simulink model "workshop_stateflow"  (R2020a)
settings: Solver=VariableStepAuto  StartTime=0.0  StopTime=inf  RelTol=1e-3
settings Model: Creator=matas  LastModifiedBy=matas

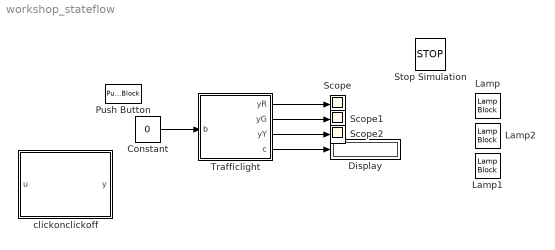
== system workshop_stateflow ==
  Constant : Constant  Value=0
  Display : Display
  Lamp : LampBlock
  Lamp1 : LampBlock
  Lamp2 : LampBlock
  Push Button : PushButtonBlock
  Scope : Scope
  Scope1 : Scope
  Scope2 : Scope
  Stop Simulation : Stop
  Trafficlight : Stateflow chart  TreatAsAtomicUnit=on
  clickonclickoff : Stateflow chart  TreatAsAtomicUnit=on
  wires:
  Constant/1 -> Trafficlight/1(b)
  Trafficlight/1(yR) -> Scope/1
  Trafficlight/2(yG) -> Scope1/1
  Trafficlight/3(yY) -> Scope2/1
  Trafficlight/4(c) -> Display/1

== stateflow chart workshop_stateflow/clickonclickoff ==
  settings: updateMethod=DISCRETE  sampleTime=0.1
  state ready_OFF
  state just_ON
  state just_OFF
  state ready_ON
  ready_OFF -> just_ON : [u==1]{y=1}
  (default) -> ready_OFF : {y=0}
  just_OFF -> ready_OFF : [u==0]{y=0}
  just_ON -> ready_OFF [commented out] : [u==0]{y=0}
  just_ON -> ready_ON : [u==0]{y=1}
  ready_ON -> just_OFF : [u==1]{y=0}
  data: u input; y output

== stateflow chart workshop_stateflow/Trafficlight ==
  settings: updateMethod=DISCRETE  sampleTime=0.1
  state Green
    during:
    c=c+1;
  state Red
    during:
    c=c+1;
  state Wait
    during:
    c=c+1;
  state Yellow
    during:
    c=c+1;
  (default) -> Red : { yR=0;
      | yY =0;
      | yG =0;
      | c=0; }
  Green -> Wait [order 2] : [(b==1)&&(c<60)]
  Red -> Green : [c==30]
      | {yR =0;
      | yG=1;
      | c=0;}
  Green -> Yellow [order 1] : [(b==1)&&(c>=60)]
      | {yG=0;
      | yY=1;
      | c=0;}
  Yellow -> Red : [c==5]
      | {yY=0;
      | yR=1;
      | c=0;}
  Wait -> Yellow : [c==60]
      | {yG=0;
      | yY=1;
      | c=0;}
  data: b input; yR output; yG output; yY output double; c output
